simulink model "nominal_tracking_REALTIME"  (R2020b)
settings: Solver=VariableStepAuto  StartTime=0.0  StopTime=10.0  RelTol=1e-3
values from neighbouring files (symbols this model uses):
  denHw = [0.03 0 0 0]    [data_v2_500.mat]    (also in data_v6_nominaldrift500.mat)
  denLPFz = [1 -0.978482055734]    [data_v2_500.mat]    (also in data_v6_nominaldrift500.mat)
  drv =     [data_v2_500.mat]    (also in data_v6_nominaldrift500.mat)
  gbox =     [data_v2_500.mat]    (also in data_v6_nominaldrift500.mat)
  N_u = 0    [data_v2_500.mat]    (also in data_v6_nominaldrift500.mat)
  N_x = [1 0 0 0]    [data_v2_500.mat]    (also in data_v6_nominaldrift500.mat)
  numHw = [1 0 0 -1]    [data_v2_500.mat]    (also in data_v6_nominaldrift500.mat)
  numLPFz = [0.0215179442657 0]    [data_v2_500.mat]    (also in data_v6_nominaldrift500.mat)
  sens =     [data_v2_500.mat]    (also in data_v6_nominaldrift500.mat)
  step_disturbance = 114.864864865    [data_v2_500.mat]    (also in data_v6_nominaldrift500.mat)
  step_size = 168.516998568    [data_v2_500.mat]    (also in data_v6_nominaldrift500.mat)
  Ts = 0.01    [data_v2_500.mat]    (also in data_v6_nominaldrift500.mat)
undefined symbols (not defined in the file or in its folder): C_gain, DiscIntNeverNeededParam, T
settings Model: Creator=39345  LastModifiedBy=39345

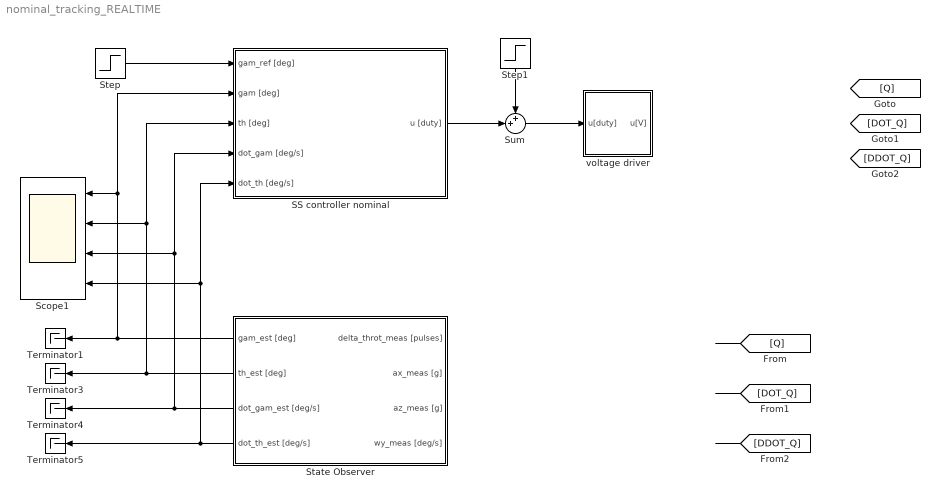
== system nominal_tracking_REALTIME ==
  SS controller nominal : Subsystem
  Scope1 : Scope  NumInputPorts=4
  State Observer : Subsystem
  Step : Step  After=step_size  SampleTime=Ts
  Step1 : Step  Time=11  After=step_disturbance  SampleTime=0.01
  Sum : Sum  Inputs=++|
  Terminator{1,3..5} (4 alike) : Terminator
  voltage driver : Subsystem
  wires:
  ? -> [DDOT_Q]
  ? -> [Q]
  Sum/1 -> voltage driver/1(u[duty])
  State Observer/4(dot_th_est [deg/s]) -> Terminator5/1, SS controller nominal/5(dot_th [deg/s]), Scope1/4
  [Q] -> ?
  [DOT_Q] -> ?
  ? -> [DOT_Q]
  State Observer/3(dot_gam_est [deg/s]) -> Terminator4/1, SS controller nominal/4(dot_gam [deg/s]), Scope1/3
  ? -> State Observer/4(wy_meas [deg/s])
  State Observer/1(gam_est [deg]) -> Terminator1/1, SS controller nominal/2(gam [deg]), Scope1/1
  Step/1 -> SS controller nominal/1(gam_ref [deg])
  Step1/1 -> Sum/1
  State Observer/2(th_est [deg]) -> Terminator3/1, SS controller nominal/3(th [deg]), Scope1/2
  ? -> State Observer/2("ax_meas [g] ")
  ? -> State Observer/1("delta_throt_meas [pulses] ")
  ? -> State Observer/3("az_meas [g] ")
  [DDOT_Q] -> ?
  SS controller nominal/1(u [duty]) -> Sum/2

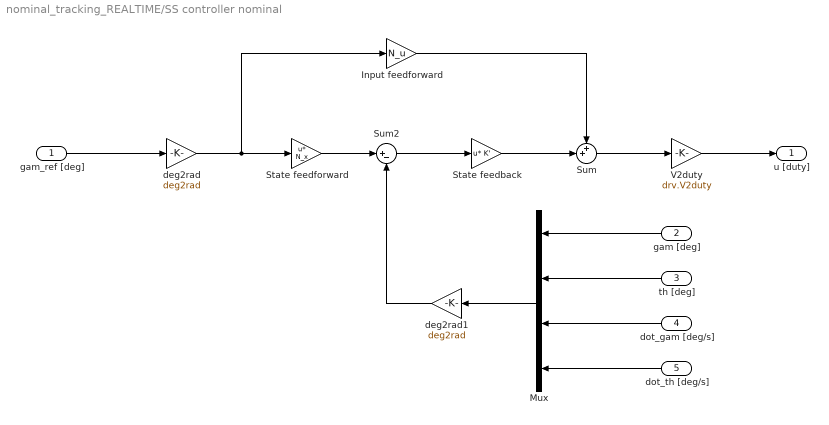
== system nominal_tracking_REALTIME/SS controller nominal ==
  gam_ref [deg] : Inport
  gam [deg] : Inport  Port=2
  th [deg] : Inport  Port=3
  dot_gam [deg/s] : Inport  Port=4
  dot_th [deg/s] : Inport  Port=5
  Input feedforward : Gain  Gain=N_u
  Mux : Mux
  State feedback : Gain  Gain=K'  Multiplication=Matrix(u*K)
  "State feedforward\t" : Gain  Gain=N_x  Multiplication=Matrix(u*K)
  Sum : Sum  Inputs=++|
  Sum2 : Sum  Inputs=|+-
  V2duty : Gain  Gain=drv.V2duty
  deg2rad : Gain  Gain=deg2rad
  deg2rad1 : Gain  Gain=deg2rad
  u [duty] : Outport
  wires:
  gam_ref [deg]/1 -> deg2rad/1
  deg2rad/1 -> Input feedforward/1, "State feedforward\t"/1
  State feedback/1 -> Sum/2
  "State feedforward\t"/1 -> Sum2/1
  Sum2/1 -> State feedback/1
  Input feedforward/1 -> Sum/1
  Sum/1 -> V2duty/1
  V2duty/1 -> u [duty]/1
  gam [deg]/1 -> Mux/1
  Mux/1 -> deg2rad1/1
  dot_gam [deg/s]/1 -> Mux/3
  th [deg]/1 -> Mux/2
  dot_th [deg/s]/1 -> Mux/4
  deg2rad1/1 -> Sum2/2

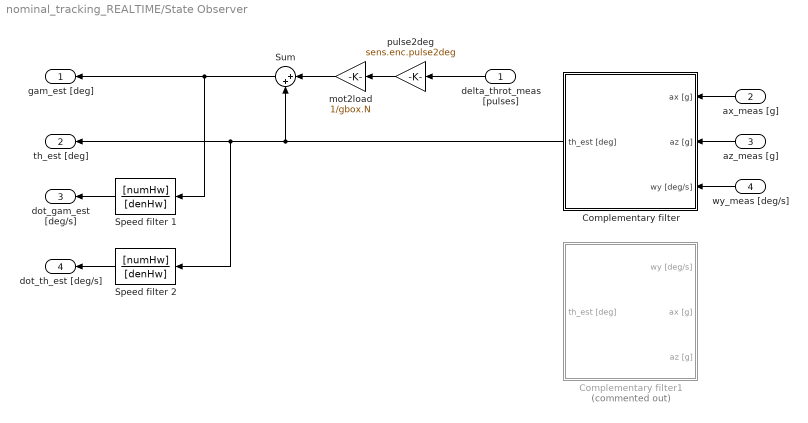
== system nominal_tracking_REALTIME/State Observer ==
  "delta_throt_meas [pulses] " : Inport
  "ax_meas [g] " : Inport  Port=2
  "az_meas [g] " : Inport  Port=3
  wy_meas [deg/s] : Inport  Port=4
  Complementary filter : Subsystem
  Complementary filter1 : Subsystem  Commented=on
  Speed filter 1 : DiscreteTransferFcn  Numerator=[numHw]  Denominator=[denHw]  SampleTime=Ts
  Speed filter 2 : DiscreteTransferFcn  Numerator=[numHw]  Denominator=[denHw]  SampleTime=Ts
  Sum : Sum  Inputs=|++
  mot2load : Gain  Gain=1/gbox.N
  pulse2deg : Gain  Gain=sens.enc.pulse2deg
  gam_est [deg] : Outport
  th_est [deg] : Outport  Port=2
  dot_gam_est [deg/s] : Outport  Port=3
  dot_th_est [deg/s] : Outport  Port=4
  wires:
  pulse2deg/1 -> mot2load/1
  "delta_throt_meas [pulses] "/1 -> pulse2deg/1
  mot2load/1 -> Sum/1
  Complementary filter/1("th_est [deg] ") -> Sum/2, Speed filter 2/1, th_est [deg]/1
  Sum/1 -> Speed filter 1/1, gam_est [deg]/1
  Speed filter 1/1 -> dot_gam_est [deg/s]/1
  Speed filter 2/1 -> dot_th_est [deg/s]/1
  "ax_meas [g] "/1 -> Complementary filter/1("ax [g] ")
  "az_meas [g] "/1 -> Complementary filter/2("az [g] ")
  wy_meas [deg/s]/1 -> Complementary filter/3(wy [deg/s])

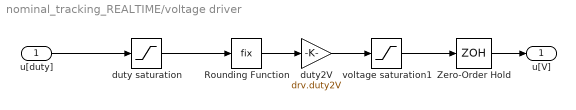
== system nominal_tracking_REALTIME/voltage driver ==
  u[duty] : Inport
  Rounding Function : Rounding  Operator=fix
  Zero-Order Hold : ZeroOrderHold  SampleTime=Ts
  duty saturation : Saturate  UpperLimit=drv.dutymax  LowerLimit=-drv.dutymax
  duty2V : Gain  Gain=drv.duty2V
  voltage saturation1 : Saturate  UpperLimit=drv.Vbus  LowerLimit=-drv.Vbus
  u[V] : Outport
  wires:
  u[duty]/1 -> duty saturation/1
  duty saturation/1 -> Rounding Function/1
  Rounding Function/1 -> duty2V/1
  duty2V/1 -> voltage saturation1/1
  voltage saturation1/1 -> Zero-Order Hold/1
  Zero-Order Hold/1 -> u[V]/1

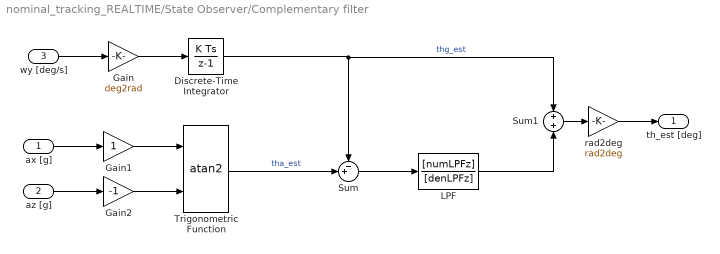
== system nominal_tracking_REALTIME/State Observer/Complementary filter ==
  "ax [g] " : Inport
  "az [g] " : Inport  Port=2
  wy [deg/s] : Inport  Port=3
  Discrete-Time Integrator : DiscreteIntegrator  gainval=1  SampleTime=Ts  ICPrevOutput=DiscIntNeverNeededParam  ICPrevScaledInput=DiscIntNeverNeededParam
  Gain : Gain  Gain=deg2rad
  Gain1 : Gain
  Gain2 : Gain  Gain=-1
  LPF : DiscreteTransferFcn  Numerator=[numLPFz]  Denominator=[denLPFz]  SampleTime=Ts
  Sum : Sum  Inputs=-+|
  Sum1 : Sum
  Trigonometric Function : Trigonometry  Operator=atan2
  rad2deg : Gain  Gain=rad2deg
  "th_est [deg] " : Outport
  wires:
  "az [g] "/1 -> Gain2/1
  "ax [g] "/1 -> Gain1/1
  wy [deg/s]/1 -> Gain/1
  Gain/1 -> Discrete-Time Integrator/1
  Gain2/1 -> Trigonometric Function/2
  Gain1/1 -> Trigonometric Function/1
  Trigonometric Function/1 -> Sum/2  "tha_est"
  Discrete-Time Integrator/1 -> Sum1/1, Sum/1  "thg_est"
  rad2deg/1 -> "th_est [deg] "/1
  Sum1/1 -> rad2deg/1
  Sum/1 -> LPF/1
  LPF/1 -> Sum1/2

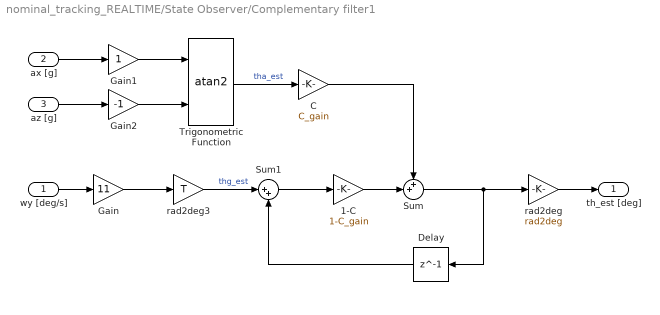
== system nominal_tracking_REALTIME/State Observer/Complementary filter1 ==
  wy [deg/s] : Inport
  "ax [g] " : Inport  Port=2
  "az [g] " : Inport  Port=3
  1-C : Gain  Gain=1-C_gain
  C : Gain  Gain=C_gain
  Delay : Delay  DelayLength=1
  Gain : Gain  Gain=11
  Gain1 : Gain
  Gain2 : Gain  Gain=-1
  Sum : Sum  Inputs=++|
  Sum1 : Sum  Inputs=|++
  Trigonometric Function : Trigonometry  Operator=atan2
  rad2deg : Gain  Gain=rad2deg
  rad2deg3 : Gain  Gain=T
  "th_est [deg] " : Outport
  wires:
  "az [g] "/1 -> Gain2/1
  "ax [g] "/1 -> Gain1/1
  wy [deg/s]/1 -> Gain/1
  Gain/1 -> rad2deg3/1
  Gain2/1 -> Trigonometric Function/2
  Gain1/1 -> Trigonometric Function/1
  rad2deg/1 -> "th_est [deg] "/1
  Trigonometric Function/1 -> C/1  "tha_est"
  C/1 -> Sum/1
  1-C/1 -> Sum/2
  Sum/1 -> Delay/1, rad2deg/1
  Delay/1 -> Sum1/2
  rad2deg3/1 -> Sum1/1  "thg_est"
  Sum1/1 -> 1-C/1
